simulink model "Linear_Decoupled_HD"  (R2022a)
settings: Solver=VariableStepAuto  StartTime=0  StopTime=1000  RelTol=1e-3
undefined symbols (not defined in the file): A_HD, A_platform, B_HD, B_platform, C_HD, C_platform, HD_op
libraries: eeGeneralControl x1
settings Model: Creator=ianam  LastModifiedBy=ianam
settings DebuggingCC: UnderSpecifiedDataTypeMsg=error  UnderSpecifiedDimensionMsg=error

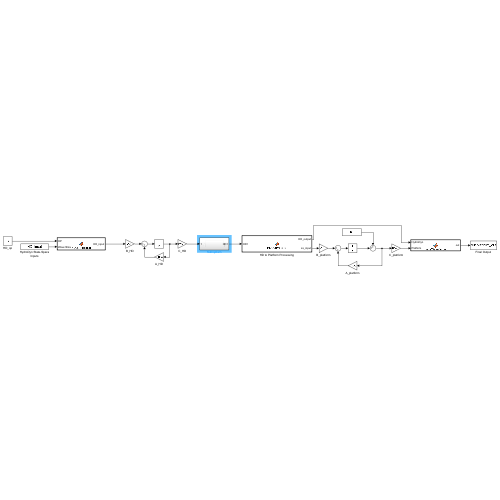
[thumbnail: Simulink's stored preview of the top-level diagram]
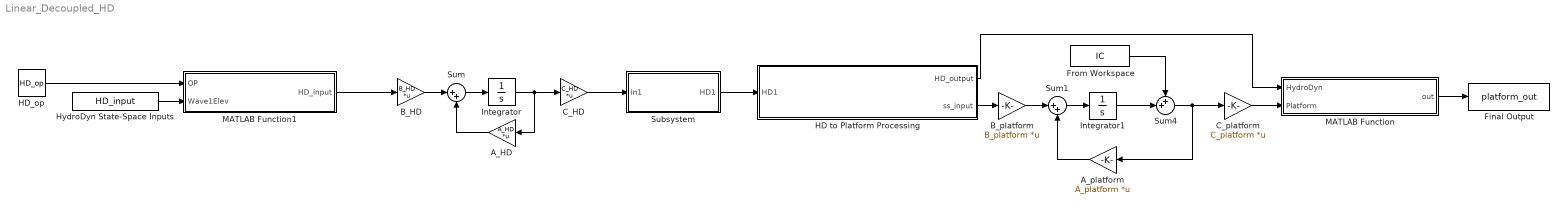
== system Linear_Decoupled_HD ==
  A_HD : Gain  Gain=A_HD  Multiplication=Matrix(K*u)
  A_platform : Gain  Gain=A_platform  Multiplication=Matrix(K*u)
  B_HD : Gain  Gain=B_HD  Multiplication=Matrix(K*u)
  B_platform : Gain  Gain=B_platform  Multiplication=Matrix(K*u)
  C_HD : Gain  Gain=C_HD  Multiplication=Matrix(K*u)
  C_platform : Gain  Gain=C_platform  Multiplication=Matrix(K*u)
  Final Output : ToWorkspace  VariableName=platform_out  SaveFormat=Timeseries  SampleTime=-1
  From Workspace : FromWorkspace  VariableName=IC
  HD to Platform Processing : MATLAB Function  TreatAsAtomicUnit=on
  HD_op : Constant  Value=HD_op
  HydroDyn State-Space Inputs : FromWorkspace  VariableName=HD_input
  Integrator : Integrator
  Integrator1 : Integrator
  MATLAB Function : MATLAB Function  TreatAsAtomicUnit=on
  MATLAB Function1 : MATLAB Function  TreatAsAtomicUnit=on
  Subsystem : Subsystem
  Sum : Sum  Inputs=|++
  Sum1 : Sum  Inputs=|++
  Sum4 : Sum  Inputs=++|
  wires:
  Sum/1 -> Integrator/1
  Integrator/1 -> C_HD/1, A_HD/1
  A_HD/1 -> Sum/2
  B_HD/1 -> Sum/1
  B_platform/1 -> Sum1/1
  Sum1/1 -> Integrator1/1
  A_platform/1 -> Sum1/2
  MATLAB Function1/1(HD_input) -> B_HD/1
  HD_op/1 -> MATLAB Function1/1(OP)
  HD to Platform Processing/2(ss_input) -> B_platform/1
  Sum4/1 -> A_platform/1, C_platform/1
  Integrator1/1 -> Sum4/2
  From Workspace/1 -> Sum4/1
  MATLAB Function/1(out) -> Final Output/1
  C_platform/1 -> MATLAB Function/2(Platform)
  HD to Platform Processing/1(HD_output) -> MATLAB Function/1(HydroDyn)
  HydroDyn State-Space Inputs/1 -> MATLAB Function1/2(Wave1Elev)
  C_HD/1 -> Subsystem/1(In1)
  Subsystem/1(HD1) -> HD to Platform Processing/1(HD1)

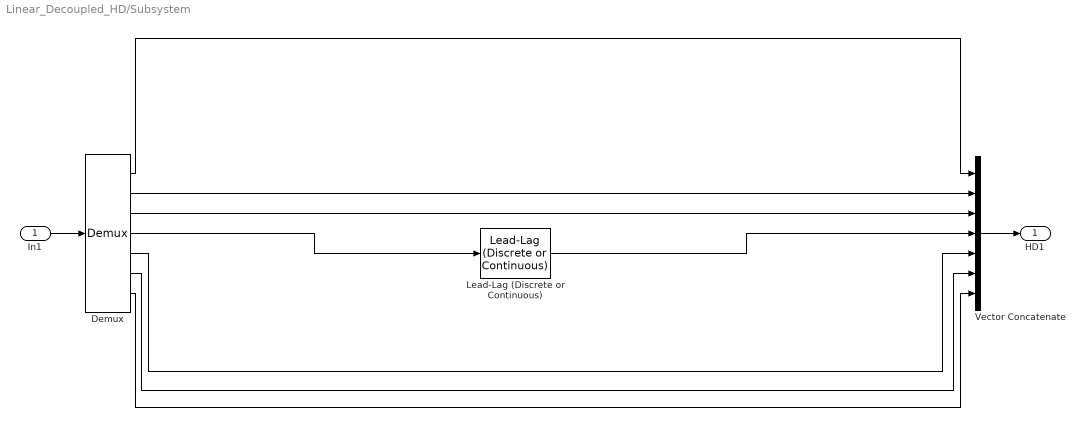
== system Linear_Decoupled_HD/Subsystem ==
  In1 : Inport
  Demux : Demux  Outputs=7
      settings: DisplayOption=none
  Lead-Lag (Discrete or Continuous) : eeGeneralControl/Lead-Lag (Discrete or Continuous)  T1=0.2  T2=0.1  B=inf  A=-inf  init_option=Inherited from block input  x0=0  Ts=-1
      settings: SourceProductBaseCode=PS
  Vector Concatenate : Concatenate  NumInputs=7
  HD1 : Outport
  wires:
  In1/1 -> Demux/1
  Vector Concatenate/1 -> HD1/1
  Demux/1 -> Vector Concatenate/1
  Demux/2 -> Vector Concatenate/2
  Demux/3 -> Vector Concatenate/3
  Demux/5 -> Vector Concatenate/5
  Demux/6 -> Vector Concatenate/6
  Demux/7 -> Vector Concatenate/7
  Demux/4 -> Lead-Lag (Discrete or Continuous)/1
  Lead-Lag (Discrete or Continuous)/1 -> Vector Concatenate/4

== matlab function Linear_Decoupled_HD/MATLAB Function1 ==
  data: OP input; Wave1Elev input; HD_input output
function HD_input = HDOutProcess(OP,Wave1Elev)

% Define quantities
% wam_trans = states(1:6);
% wam_vel = states(11:16);

% Create input vector
HD_input = zeros(37,1);

% Assign HD outputs to input vector
% HD_input(1:6) = wam_trans;
% HD_input(7:12) = wam_vel;
HD_input(37) = Wave1Elev;

% Add operating point to inputs
HD_input = HD_input + OP;

end

== matlab function Linear_Decoupled_HD/HD to Platform Processing ==
  data: HD_output output; HD1 input; ss_input output size=235,1
function [HD_output,ss_input] = HDOutProcess(HD1)

% Initialize
HydroF = zeros(6,1);
HD_output = zeros(25,1);

% Define quantities
Wave1Elev = HD1(1);
HydroF(1) = HD1(2);
HydroF(2) = HD1(3);
HydroF(3) = HD1(4);
HydroF(4) = HD1(5);
HydroF(5) = HD1(6);
HydroF(6) = HD1(7);

HD_output(:,1) = HD1(:);
HD_output(2:7) = HD_output(2:7);
HD_output(8:13) = HD_output(8:13);

% Create input vector
ss_input = zeros(235,1);

% Assign HD outputs to input vector
ss_input(40:45,1) = HydroF(:,1);

ss_input(226,1) = Wave1Elev(1);

end

== matlab function Linear_Decoupled_HD/MATLAB Function ==
  data: HydroDyn input; out output; Platform input
function out = passWaveForce(HydroDyn,Platform)

% Read Forces from HydroDyn Output
force = HydroDyn(2:end,1);

% Add Forces to Total Output
Platform(34:57,1) = force;

out = Platform;

end
